simulink model "SimunlikReferenceDiffWindowSizes"  (R2021b)
settings: Solver=VariableStepAuto  StartTime=0.0  StopTime=2048*15/fs  RelTol=1e-3
InitFcn:
  | f = 12.288e6;
  | fs = 153.6e6;
  | N1 = 256;
  | N2 = 512;
  | N3 = 1024;
  | N4 = 2048;
  | N5 = 4096;
  | n1 = 0:N1-1;
  | n2 = 0:N2-1;
  | n3 = 0:N3-1;
  | n4 = 0:N4-1;
  | n5 = 0:N5-1;
  | Hamming1 = 0.54 - 0.46 * cos(2*pi*n1/N1);
  | Hamming2 = 0.54 - 0.46 * cos(2*pi*n2/N2);
  | Hamming3 = 0.54 - 0.46 * cos(2*pi*n3/N3);
  | Hamming4 = 0.54 - 0.46 * cos(2*pi*n4/N4);
  | Hamming5 = 0.54 - 0.46 * cos(2*pi*n5/N5);
  | Hanning1 = 0.5 * (1 + cos(2*pi*n1/N1));
  | Hanning2 = 0.5 * (1 + cos(2*pi*n2/N2));
  | Hanning3 = 0.5 * (1 + cos(2*pi*n3/N3));
  | Hanning4 = 0.5 * (1 + cos(2*pi*n4/N4));
  | Hanning5 = 0.5 * (1 + cos(2*pi*n5/N5));
  | Norm_Ham1 = sum(Hamming1);
  | Norm_Ham2 = sum(Hamming2);
  | Norm_Ham3 = sum(Hamming3);
  | Norm_Ham4 = sum(Hamming4);
  | Norm_Ham5 = sum(Hamming5);
  | Norm_Han1 = sum(Hanning1);
  | Norm_Han2 = sum(Hanning2);
  | Norm_Han3 = sum(Hanning3);
  | Norm_Han4 = sum(Hanning4);
  | Norm_Han5 = sum(Hanning5);
undefined symbols (not defined in the file): AXI4, Lite
libraries: dspxfrm3 x10, dspsigops x10, hdlBasic x7, hdlsllib x1, vmcUtilities x1
settings Model: Creator=yxb20126  LastModifiedBy=yxb20126

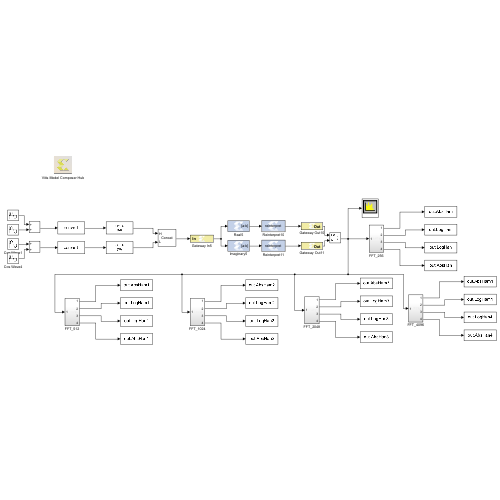
[thumbnail: Simulink's stored preview of the top-level diagram]
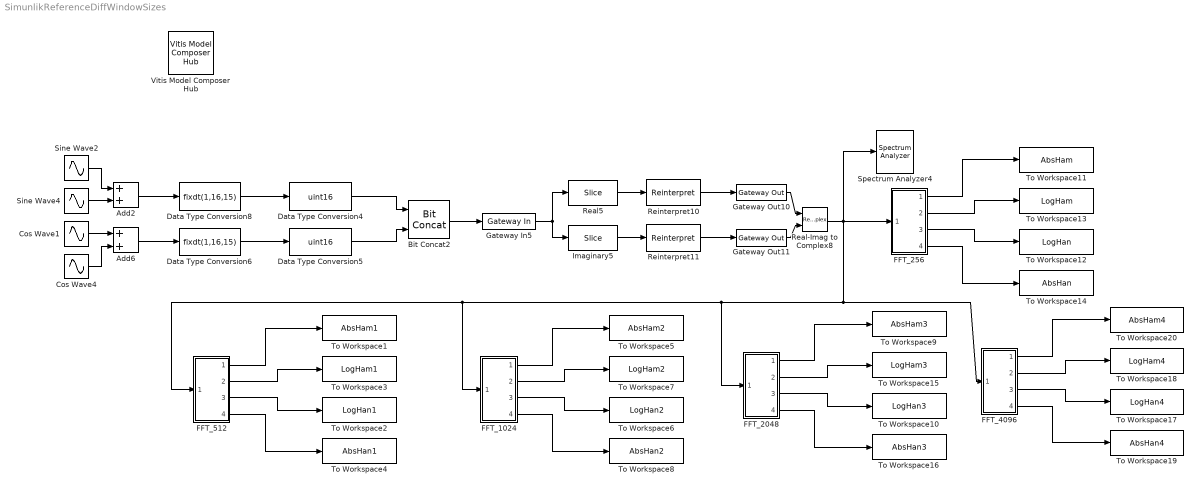
== system SimunlikReferenceDiffWindowSizes ==
  Add2 : Sum
  Add6 : Sum
  Bit Concat2 : hdlsllib/Logic and Bit Operations/Bit Concat  numInputs=2
  Cos Wave1 : Sin  Amplitude=0.4  Frequency=f*2*pi  Phase=pi/2  SampleTime=1/fs
  Cos Wave4 : Sin  Amplitude=0.4  Frequency=f*pi  Phase=pi/2  SampleTime=1/fs
  Data Type Conversion4 : DataTypeConversion  OutDataTypeStr=uint16  ConvertRealWorld=Stored Integer (SI)
  Data Type Conversion5 : DataTypeConversion  OutDataTypeStr=uint16  ConvertRealWorld=Stored Integer (SI)
  Data Type Conversion6 : DataTypeConversion  OutDataTypeStr=fixdt(1,16,15)  SaturateOnIntegerOverflow=on
  Data Type Conversion8 : DataTypeConversion  OutDataTypeStr=fixdt(1,16,15)  SaturateOnIntegerOverflow=on
  FFT_1024 : Subsystem
  FFT_2048 : Subsystem
  FFT_256 : Subsystem
  FFT_4096 : Subsystem
  FFT_512 : Subsystem
  Gateway In5 : hdlBasic/Gateway In  gui_display_data_type=Fixed-point  arith_type=Unsigned  n_bits=32  bin_pt=0  preci_type=Single  exp_width=8  frac_width=24  rows=1  columns=1  quantization=Truncate  overflow=Wrap  period=1/fs  UseAsADC=off  ADCChannel='1'  interface=AXI4-Lite  automatic_assignment=on  address_offset=hex2dec('00')  intf_name=''  intf_description=''  default_value=0  timing_constraint=None  locs_specified=off  LOCs={}  io_standard={}  inherit_from_input=off  hdl_port=on  XmcBlockStatus=1  maskContainerNames=group4  block_type=gatewayin  block_config=sysgen:gateway_in_config  block_width_w=590  block_height_w=620  block_width=640  block_height=850
  Gateway Out10 : hdlBasic/Gateway Out  inherit_from_input=off  hdl_port=on  rows=1  columns=1  UseAsDAC=off  DACChannel='1'  interface=AXI4-Lite  automatic_assignment=on  address_offset=hex2dec('00')  intf_name=''  intf_description=''  timing_constraint=None  locs_specified=off  LOCs={}  io_standard={}  XmcBlockStatus=1  maskContainerNames=group4  block_type=gatewayout  block_config=sysgen:gateway_out_config  block_width_w=590  block_height_w=620  block_width=620  block_height=750
  Gateway Out11 : hdlBasic/Gateway Out  inherit_from_input=off  hdl_port=on  rows=1  columns=1  UseAsDAC=off  DACChannel='1'  interface=AXI4-Lite  automatic_assignment=on  address_offset=hex2dec('00')  intf_name=''  intf_description=''  timing_constraint=None  locs_specified=off  LOCs={}  io_standard={}  XmcBlockStatus=1  maskContainerNames=group4  block_type=gatewayout  block_config=sysgen:gateway_out_config  block_width_w=590  block_height_w=620  block_width=620  block_height=750
  Imaginary5 : hdlBasic/Slice  nbits=16  boolean_output=off  mode=Two Bit Locations  bit1=31  base1=LSB of Input  bit0=16  base0=LSB of Input  XmcBlockStatus=1  maskContainerNames=group1  block_type=slice  block_config=sysgen:Slice_config
  Real-Imag to Complex8 : RealImagToComplex
  Real5 : hdlBasic/Slice  nbits=16  boolean_output=off  mode=Two Bit Locations  bit1=15  base1=LSB of Input  bit0=0  base0=LSB of Input  XmcBlockStatus=1  maskContainerNames=group1  block_type=slice  block_config=sysgen:Slice_config
  Reinterpret10 : hdlBasic/Reinterpret  force_arith_type=on  arith_type="Signed  (2's comp)"  force_bin_pt=off  bin_pt=0  XmcBlockStatus=1  maskContainerNames=group1  block_type=reinterpret  block_config=sysgen:Reinterpret_config
  Reinterpret11 : hdlBasic/Reinterpret  force_arith_type=on  arith_type="Signed  (2's comp)"  force_bin_pt=off  bin_pt=0  XmcBlockStatus=1  maskContainerNames=group1  block_type=reinterpret  block_config=sysgen:Reinterpret_config
  Sine Wave2 : Sin  Amplitude=0.4  Frequency=f*2*pi  SampleTime=1/fs
  Sine Wave4 : Sin  Amplitude=0.4  Frequency=f*pi  SampleTime=1/fs
  Spectrum Analyzer4 : SpectrumAnalyzer
  To Workspace1 : ToWorkspace  VariableName=AbsHam1  SampleTime=-1
      settings: Save2DSignal=2-D array (concatenate along first dimension)
  To Workspace10 : ToWorkspace  VariableName=LogHan3  SampleTime=-1
      settings: Save2DSignal=2-D array (concatenate along first dimension)
  To Workspace11 : ToWorkspace  VariableName=AbsHam  SampleTime=-1
      settings: Save2DSignal=2-D array (concatenate along first dimension)
  To Workspace12 : ToWorkspace  VariableName=LogHan  SampleTime=-1
      settings: Save2DSignal=2-D array (concatenate along first dimension)
  To Workspace13 : ToWorkspace  VariableName=LogHam  SampleTime=-1
      settings: Save2DSignal=2-D array (concatenate along first dimension)
  To Workspace14 : ToWorkspace  VariableName=AbsHan  SampleTime=-1
      settings: Save2DSignal=2-D array (concatenate along first dimension)
  To Workspace15 : ToWorkspace  VariableName=LogHam3  SampleTime=-1
      settings: Save2DSignal=2-D array (concatenate along first dimension)
  To Workspace16 : ToWorkspace  VariableName=AbsHan3  SampleTime=-1
      settings: Save2DSignal=2-D array (concatenate along first dimension)
  To Workspace17 : ToWorkspace  VariableName=LogHan4  SampleTime=-1
      settings: Save2DSignal=2-D array (concatenate along first dimension)
  To Workspace18 : ToWorkspace  VariableName=LogHam4  SampleTime=-1
      settings: Save2DSignal=2-D array (concatenate along first dimension)
  To Workspace19 : ToWorkspace  VariableName=AbsHan4  SampleTime=-1
      settings: Save2DSignal=2-D array (concatenate along first dimension)
  To Workspace2 : ToWorkspace  VariableName=LogHan1  SampleTime=-1
      settings: Save2DSignal=2-D array (concatenate along first dimension)
  To Workspace20 : ToWorkspace  VariableName=AbsHam4  SampleTime=-1
      settings: Save2DSignal=2-D array (concatenate along first dimension)
  To Workspace3 : ToWorkspace  VariableName=LogHam1  SampleTime=-1
      settings: Save2DSignal=2-D array (concatenate along first dimension)
  To Workspace4 : ToWorkspace  VariableName=AbsHan1  SampleTime=-1
      settings: Save2DSignal=2-D array (concatenate along first dimension)
  To Workspace5 : ToWorkspace  VariableName=AbsHam2  SampleTime=-1
      settings: Save2DSignal=2-D array (concatenate along first dimension)
  To Workspace6 : ToWorkspace  VariableName=LogHan2  SampleTime=-1
      settings: Save2DSignal=2-D array (concatenate along first dimension)
  To Workspace7 : ToWorkspace  VariableName=LogHam2  SampleTime=-1
      settings: Save2DSignal=2-D array (concatenate along first dimension)
  To Workspace8 : ToWorkspace  VariableName=AbsHan2  SampleTime=-1
      settings: Save2DSignal=2-D array (concatenate along first dimension)
  To Workspace9 : ToWorkspace  VariableName=AbsHam3  SampleTime=-1
      settings: Save2DSignal=2-D array (concatenate along first dimension)
  Vitis Model Composer Hub : vmcUtilities/Vitis Model Composer Hub  Tag=genX  CodeGeneration=off  SubsystemName=<enter or select subsystem name>  TargetDirectory=./code  ExportType=HLS C++ code  IpVendor=xilinx.com  IpLibrary=hls  IpVersion=1.0  IpHWLanguage=Verilog  AieCompilerOptions={}  CreateTestbench=off  TestbenchStackSize=10  RunAieSim=off  AieSimTimeout=50000  RunAieSimProfiling=off  LaunchVitisAnalyzer=off  PlotOutput=off  RunX86Sim=off  X86SimTimeout=10  GenHwImage=off  PlatformType=Not Specified  HwSystemType=Baremetal  HwValidationTarget=hw  ProjDevice=xczu48dr-ffvg1517-2-e  ProjDevicePart=xczu48dr-ffvg1517-2-e  SamplePeriod=-1  ClockFrequency=200  DataPathParallelism=1  xilinxfamily=zynquplusRFSOC  part=xczu48dr  speed=-2-e  package=ffvg1517  directory=./netlist  testbench=off  incr_netlist=off  synthesis_tool=Vivado  clock_wrapper=Clock Enables  dbl_ovrd=According to Block Masks  dcm_input_clock_period=10  sysclk_period=(1/fs)*10e9  simulink_period=1/fs  eval_field=0
  wires:
  FFT_256/1(Out1) -> To Workspace11/1
  FFT_256/2(Out2) -> To Workspace13/1
  Gateway Out10/1 -> Real-Imag to Complex8/1
  FFT_256/4(Out4) -> To Workspace14/1
  FFT_256/3(Out3) -> To Workspace12/1
  Reinterpret11/1 -> Gateway Out11/1
  Real-Imag to Complex8/1 -> FFT_4096/1(In1), FFT_2048/1(In1), FFT_1024/1(In1), FFT_512/1(In1), FFT_256/1(In1), Spectrum Analyzer4/1
  Gateway In5/1 -> Imaginary5/1, Real5/1
  Imaginary5/1 -> Reinterpret11/1
  Reinterpret10/1 -> Gateway Out10/1
  Gateway Out11/1 -> Real-Imag to Complex8/2
  Real5/1 -> Reinterpret10/1
  FFT_512/3(Out3) -> To Workspace2/1
  FFT_512/4(Out4) -> To Workspace4/1
  FFT_512/2(Out2) -> To Workspace3/1
  FFT_512/1(Out1) -> To Workspace1/1
  FFT_1024/1(Out1) -> To Workspace5/1
  FFT_1024/2(Out2) -> To Workspace7/1
  FFT_1024/4(Out4) -> To Workspace8/1
  FFT_1024/3(Out3) -> To Workspace6/1
  FFT_2048/3(Out3) -> To Workspace10/1
  FFT_2048/4(Out4) -> To Workspace16/1
  FFT_2048/2(Out2) -> To Workspace15/1
  FFT_2048/1(Out1) -> To Workspace9/1
  FFT_4096/1(Out1) -> To Workspace20/1
  FFT_4096/2(Out2) -> To Workspace18/1
  FFT_4096/4(Out4) -> To Workspace19/1
  FFT_4096/3(Out3) -> To Workspace17/1
  Data Type Conversion5/1 -> Bit Concat2/2
  Data Type Conversion8/1 -> Data Type Conversion4/1
  Add6/1 -> Data Type Conversion6/1
  Sine Wave4/1 -> Add2/2
  Sine Wave2/1 -> Add2/1
  Add2/1 -> Data Type Conversion8/1
  Cos Wave1/1 -> Add6/1
  Data Type Conversion6/1 -> Data Type Conversion5/1
  Data Type Conversion4/1 -> Bit Concat2/1
  Cos Wave4/1 -> Add6/2
  Bit Concat2/1 -> Gateway In5/1

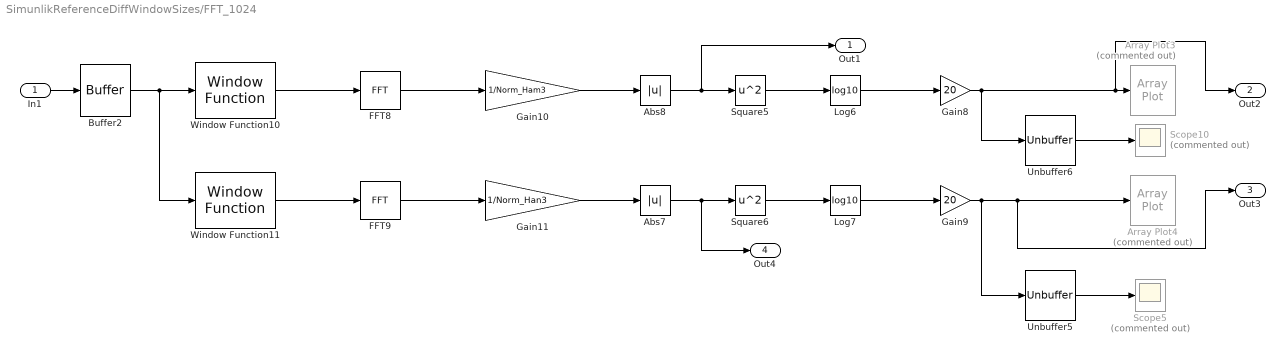
== system SimunlikReferenceDiffWindowSizes/FFT_1024 ==
  In1 : Inport
  Abs7 : Abs
  Abs8 : Abs
  Array Plot3 : ArrayPlot  Commented=on  WindowPosition=[827.000000,398.000000,581.000000,481.000000,]  YLimits=[-59.68956955456875,167.07325575587276]  ShowLegend=on
  Array Plot4 : ArrayPlot  Commented=on  WindowPosition=[214.000000,393.000000,581.000000,481.000000,]  YLimits=[-59.68956955456875,167.07325575587276]  ShowLegend=on
  Buffer2 : Buffer  N=N3  OutputFrames=off
  FFT8 : dspxfrm3/FFT  FFTImplementation=Auto  CompMethod=Table lookup  TableOpt=NEW  TableOptActive=Speed  BitRevOrder=off  Normalize=off  InheritFFTLength=off  FFTLength=N3  WrapInput=off  roundingMode=Floor  overflowMode=off  firstCoeffDataTypeStr=Inherit: Same word length as input  firstCoeffLastDataTypeStr=Inherit: Same word length as input  outputMin=[]  outputMax=[]
  FFT9 : dspxfrm3/FFT  FFTImplementation=Auto  CompMethod=Table lookup  TableOpt=NEW  TableOptActive=Speed  BitRevOrder=off  Normalize=off  InheritFFTLength=off  FFTLength=N3  WrapInput=off  roundingMode=Floor  overflowMode=off  firstCoeffDataTypeStr=Inherit: Same word length as input  firstCoeffLastDataTypeStr=Inherit: Same word length as input  outputMin=[]  outputMax=[]
  Gain10 : Gain  Gain=1/Norm_Ham3
  Gain11 : Gain  Gain=1/Norm_Han3
  Gain8 : Gain  Gain=20
  Gain9 : Gain  Gain=20
  Log6 : Math  Operator=log10  OutputSignalType=complex  SaturateOnIntegerOverflow=on
  Log7 : Math  Operator=log10  OutputSignalType=complex  SaturateOnIntegerOverflow=on
  Scope10 : Scope  Commented=on
  Scope5 : Scope  Commented=on
  Square5 : Math  Operator=square  SaturateOnIntegerOverflow=on
  Square6 : Math  Operator=square  SaturateOnIntegerOverflow=on
  Unbuffer5 : Unbuffer
  Unbuffer6 : Unbuffer
  Window Function10 : dspsigops/Window Function  winmode=Apply window to input  wintype=Hamming  sampmode=Continuous  samptime=1  N=64  Rs=50  beta=10  winsamp=Symmetric  UserWindow=hamming  OptParams=off  UserParams={'symmetric'}  dataType=double  isSigned=on  wordLen=16  udDataType=sfix(16)  fracBitsMode=Best precision  numFracBits=15  roundingMode=Floor  overflowMode=on  numSidelobes=4  sidelobeLevel=-30
      settings: SourceProductBaseCode=DS
  Window Function11 : dspsigops/Window Function  winmode=Apply window to input  wintype=Hann  sampmode=Continuous  samptime=1  N=64  Rs=50  beta=10  winsamp=Symmetric  UserWindow=hamming  OptParams=off  UserParams={'symmetric'}  dataType=double  isSigned=on  wordLen=16  udDataType=sfix(16)  fracBitsMode=Best precision  numFracBits=15  roundingMode=Floor  overflowMode=on  numSidelobes=4  sidelobeLevel=-30
      settings: SourceProductBaseCode=DS
  Out1 : Outport
  Out2 : Outport  Port=2
  Out3 : Outport  Port=3
  Out4 : Outport  Port=4
  wires:
  FFT8/1 -> Gain10/1
  Unbuffer6/1 -> Scope10/1
  Log6/1 -> Gain8/1
  Gain8/1 -> Out2/1, Array Plot3/1, Unbuffer6/1
  Square5/1 -> Log6/1
  Gain9/1 -> Out3/1, Array Plot4/1, Unbuffer5/1
  Buffer2/1 -> Window Function11/1, Window Function10/1
  Abs8/1 -> Out1/1, Square5/1
  Window Function11/1 -> FFT9/1
  Log7/1 -> Gain9/1
  Square6/1 -> Log7/1
  Window Function10/1 -> FFT8/1
  Unbuffer5/1 -> Scope5/1
  In1/1 -> Buffer2/1
  Abs7/1 -> Out4/1, Square6/1
  Gain10/1 -> Abs8/1
  Gain11/1 -> Abs7/1
  FFT9/1 -> Gain11/1

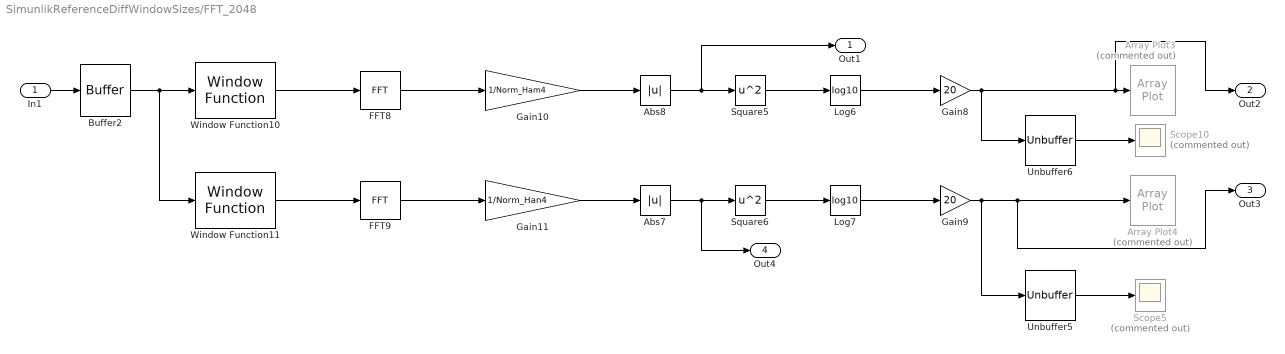
== system SimunlikReferenceDiffWindowSizes/FFT_2048 ==
  In1 : Inport
  Abs7 : Abs
  Abs8 : Abs
  Array Plot3 : ArrayPlot  Commented=on  WindowPosition=[827.000000,398.000000,581.000000,481.000000,]  YLimits=[-59.68956955456875,167.07325575587276]  ShowLegend=on
  Array Plot4 : ArrayPlot  Commented=on  WindowPosition=[214.000000,393.000000,581.000000,481.000000,]  YLimits=[-59.68956955456875,167.07325575587276]  ShowLegend=on
  Buffer2 : Buffer  N=N4  OutputFrames=off
  FFT8 : dspxfrm3/FFT  FFTImplementation=Auto  CompMethod=Table lookup  TableOpt=NEW  TableOptActive=Speed  BitRevOrder=off  Normalize=off  InheritFFTLength=off  FFTLength=N4  WrapInput=off  roundingMode=Floor  overflowMode=off  firstCoeffDataTypeStr=Inherit: Same word length as input  firstCoeffLastDataTypeStr=Inherit: Same word length as input  outputMin=[]  outputMax=[]
  FFT9 : dspxfrm3/FFT  FFTImplementation=Auto  CompMethod=Table lookup  TableOpt=NEW  TableOptActive=Speed  BitRevOrder=off  Normalize=off  InheritFFTLength=off  FFTLength=N4  WrapInput=off  roundingMode=Floor  overflowMode=off  firstCoeffDataTypeStr=Inherit: Same word length as input  firstCoeffLastDataTypeStr=Inherit: Same word length as input  outputMin=[]  outputMax=[]
  Gain10 : Gain  Gain=1/Norm_Ham4
  Gain11 : Gain  Gain=1/Norm_Han4
  Gain8 : Gain  Gain=20
  Gain9 : Gain  Gain=20
  Log6 : Math  Operator=log10  OutputSignalType=complex  SaturateOnIntegerOverflow=on
  Log7 : Math  Operator=log10  OutputSignalType=complex  SaturateOnIntegerOverflow=on
  Scope10 : Scope  Commented=on
  Scope5 : Scope  Commented=on
  Square5 : Math  Operator=square  SaturateOnIntegerOverflow=on
  Square6 : Math  Operator=square  SaturateOnIntegerOverflow=on
  Unbuffer5 : Unbuffer
  Unbuffer6 : Unbuffer
  Window Function10 : dspsigops/Window Function  winmode=Apply window to input  wintype=Hamming  sampmode=Continuous  samptime=1  N=64  Rs=50  beta=10  winsamp=Symmetric  UserWindow=hamming  OptParams=off  UserParams={'symmetric'}  dataType=double  isSigned=on  wordLen=16  udDataType=sfix(16)  fracBitsMode=Best precision  numFracBits=15  roundingMode=Floor  overflowMode=on  numSidelobes=4  sidelobeLevel=-30
      settings: SourceProductBaseCode=DS
  Window Function11 : dspsigops/Window Function  winmode=Apply window to input  wintype=Hann  sampmode=Continuous  samptime=1  N=64  Rs=50  beta=10  winsamp=Symmetric  UserWindow=hamming  OptParams=off  UserParams={'symmetric'}  dataType=double  isSigned=on  wordLen=16  udDataType=sfix(16)  fracBitsMode=Best precision  numFracBits=15  roundingMode=Floor  overflowMode=on  numSidelobes=4  sidelobeLevel=-30
      settings: SourceProductBaseCode=DS
  Out1 : Outport
  Out2 : Outport  Port=2
  Out3 : Outport  Port=3
  Out4 : Outport  Port=4
  wires:
  FFT9/1 -> Gain11/1
  Gain11/1 -> Abs7/1
  Gain10/1 -> Abs8/1
  Abs7/1 -> Square6/1, Out4/1
  In1/1 -> Buffer2/1
  Unbuffer5/1 -> Scope5/1
  Window Function10/1 -> FFT8/1
  Square6/1 -> Log7/1
  Log7/1 -> Gain9/1
  Window Function11/1 -> FFT9/1
  Abs8/1 -> Square5/1, Out1/1
  Buffer2/1 -> Window Function10/1, Window Function11/1
  Gain9/1 -> Unbuffer5/1, Array Plot4/1, Out3/1
  Square5/1 -> Log6/1
  Gain8/1 -> Unbuffer6/1, Array Plot3/1, Out2/1
  Log6/1 -> Gain8/1
  Unbuffer6/1 -> Scope10/1
  FFT8/1 -> Gain10/1

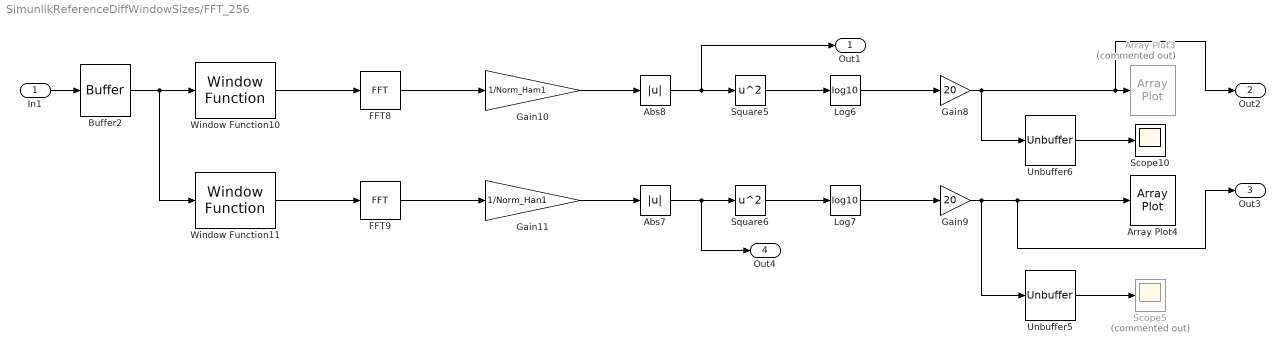
== system SimunlikReferenceDiffWindowSizes/FFT_256 ==
  In1 : Inport
  Abs7 : Abs
  Abs8 : Abs
  Array Plot3 : ArrayPlot  Commented=on  WindowPosition=[827.000000,398.000000,581.000000,481.000000,]  YLimits=[-59.68956955456875,167.07325575587276]  ShowLegend=on
  Array Plot4 : ArrayPlot  WindowPosition=[214.000000,393.000000,581.000000,481.000000,]  YLimits=[-59.68956955456875,167.07325575587276]  ShowLegend=on
  Buffer2 : Buffer  N=N1  OutputFrames=off
  FFT8 : dspxfrm3/FFT  FFTImplementation=Auto  CompMethod=Table lookup  TableOpt=NEW  TableOptActive=Speed  BitRevOrder=off  Normalize=off  InheritFFTLength=off  FFTLength=N1  WrapInput=off  roundingMode=Floor  overflowMode=off  firstCoeffDataTypeStr=Inherit: Same word length as input  firstCoeffLastDataTypeStr=Inherit: Same word length as input  outputMin=[]  outputMax=[]
  FFT9 : dspxfrm3/FFT  FFTImplementation=Auto  CompMethod=Table lookup  TableOpt=NEW  TableOptActive=Speed  BitRevOrder=off  Normalize=off  InheritFFTLength=off  FFTLength=N1  WrapInput=off  roundingMode=Floor  overflowMode=off  firstCoeffDataTypeStr=Inherit: Same word length as input  firstCoeffLastDataTypeStr=Inherit: Same word length as input  outputMin=[]  outputMax=[]
  Gain10 : Gain  Gain=1/Norm_Ham1
  Gain11 : Gain  Gain=1/Norm_Han1
  Gain8 : Gain  Gain=20
  Gain9 : Gain  Gain=20
  Log6 : Math  Operator=log10  OutputSignalType=complex  SaturateOnIntegerOverflow=on
  Log7 : Math  Operator=log10  OutputSignalType=complex  SaturateOnIntegerOverflow=on
  Scope10 : Scope
  Scope5 : Scope  Commented=on
  Square5 : Math  Operator=square  SaturateOnIntegerOverflow=on
  Square6 : Math  Operator=square  SaturateOnIntegerOverflow=on
  Unbuffer5 : Unbuffer
  Unbuffer6 : Unbuffer
  Window Function10 : dspsigops/Window Function  winmode=Apply window to input  wintype=Hamming  sampmode=Continuous  samptime=1  N=64  Rs=50  beta=10  winsamp=Symmetric  UserWindow=hamming  OptParams=off  UserParams={'symmetric'}  dataType=double  isSigned=on  wordLen=16  udDataType=sfix(16)  fracBitsMode=Best precision  numFracBits=15  roundingMode=Floor  overflowMode=on  numSidelobes=4  sidelobeLevel=-30
      settings: SourceProductBaseCode=DS
  Window Function11 : dspsigops/Window Function  winmode=Apply window to input  wintype=Hann  sampmode=Continuous  samptime=1  N=64  Rs=50  beta=10  winsamp=Symmetric  UserWindow=hamming  OptParams=off  UserParams={'symmetric'}  dataType=double  isSigned=on  wordLen=16  udDataType=sfix(16)  fracBitsMode=Best precision  numFracBits=15  roundingMode=Floor  overflowMode=on  numSidelobes=4  sidelobeLevel=-30
      settings: SourceProductBaseCode=DS
  Out1 : Outport
  Out2 : Outport  Port=2
  Out3 : Outport  Port=3
  Out4 : Outport  Port=4
  wires:
  FFT8/1 -> Gain10/1
  Unbuffer6/1 -> Scope10/1
  Log6/1 -> Gain8/1
  Gain8/1 -> Out2/1, Array Plot3/1, Unbuffer6/1
  Square5/1 -> Log6/1
  Gain9/1 -> Out3/1, Array Plot4/1, Unbuffer5/1
  Buffer2/1 -> Window Function11/1, Window Function10/1
  Abs8/1 -> Out1/1, Square5/1
  Window Function11/1 -> FFT9/1
  Log7/1 -> Gain9/1
  Square6/1 -> Log7/1
  Window Function10/1 -> FFT8/1
  Unbuffer5/1 -> Scope5/1
  In1/1 -> Buffer2/1
  Abs7/1 -> Out4/1, Square6/1
  Gain10/1 -> Abs8/1
  Gain11/1 -> Abs7/1
  FFT9/1 -> Gain11/1

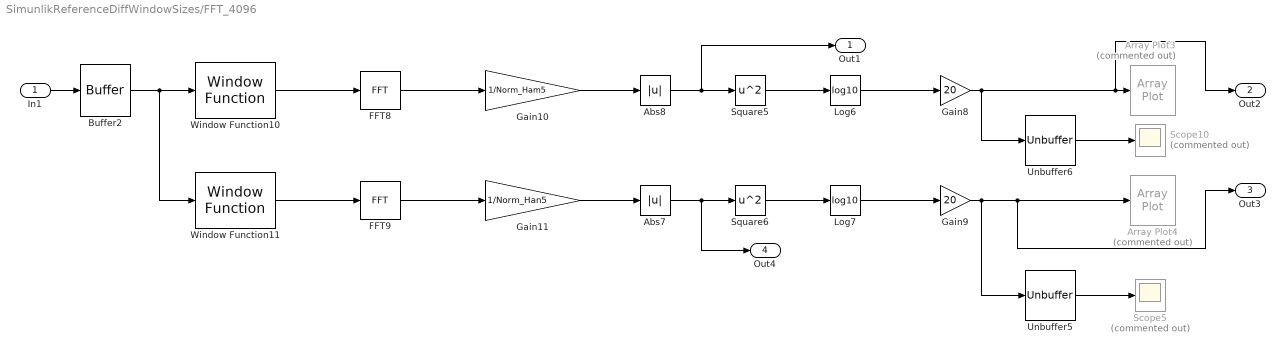
== system SimunlikReferenceDiffWindowSizes/FFT_4096 ==
  In1 : Inport
  Abs7 : Abs
  Abs8 : Abs
  Array Plot3 : ArrayPlot  Commented=on  WindowPosition=[827.000000,398.000000,581.000000,481.000000,]  YLimits=[-59.68956955456875,167.07325575587276]  ShowLegend=on
  Array Plot4 : ArrayPlot  Commented=on  WindowPosition=[214.000000,393.000000,581.000000,481.000000,]  YLimits=[-59.68956955456875,167.07325575587276]  ShowLegend=on
  Buffer2 : Buffer  N=N5  OutputFrames=off
  FFT8 : dspxfrm3/FFT  FFTImplementation=Auto  CompMethod=Table lookup  TableOpt=NEW  TableOptActive=Speed  BitRevOrder=off  Normalize=off  InheritFFTLength=off  FFTLength=N5  WrapInput=off  roundingMode=Floor  overflowMode=off  firstCoeffDataTypeStr=Inherit: Same word length as input  firstCoeffLastDataTypeStr=Inherit: Same word length as input  outputMin=[]  outputMax=[]
  FFT9 : dspxfrm3/FFT  FFTImplementation=Auto  CompMethod=Table lookup  TableOpt=NEW  TableOptActive=Speed  BitRevOrder=off  Normalize=off  InheritFFTLength=off  FFTLength=N5  WrapInput=off  roundingMode=Floor  overflowMode=off  firstCoeffDataTypeStr=Inherit: Same word length as input  firstCoeffLastDataTypeStr=Inherit: Same word length as input  outputMin=[]  outputMax=[]
  Gain10 : Gain  Gain=1/Norm_Ham5
  Gain11 : Gain  Gain=1/Norm_Han5
  Gain8 : Gain  Gain=20
  Gain9 : Gain  Gain=20
  Log6 : Math  Operator=log10  OutputSignalType=complex  SaturateOnIntegerOverflow=on
  Log7 : Math  Operator=log10  OutputSignalType=complex  SaturateOnIntegerOverflow=on
  Scope10 : Scope  Commented=on
  Scope5 : Scope  Commented=on
  Square5 : Math  Operator=square  SaturateOnIntegerOverflow=on
  Square6 : Math  Operator=square  SaturateOnIntegerOverflow=on
  Unbuffer5 : Unbuffer
  Unbuffer6 : Unbuffer
  Window Function10 : dspsigops/Window Function  winmode=Apply window to input  wintype=Hamming  sampmode=Continuous  samptime=1  N=64  Rs=50  beta=10  winsamp=Symmetric  UserWindow=hamming  OptParams=off  UserParams={'symmetric'}  dataType=double  isSigned=on  wordLen=16  udDataType=sfix(16)  fracBitsMode=Best precision  numFracBits=15  roundingMode=Floor  overflowMode=on  numSidelobes=4  sidelobeLevel=-30
      settings: SourceProductBaseCode=DS
  Window Function11 : dspsigops/Window Function  winmode=Apply window to input  wintype=Hann  sampmode=Continuous  samptime=1  N=64  Rs=50  beta=10  winsamp=Symmetric  UserWindow=hamming  OptParams=off  UserParams={'symmetric'}  dataType=double  isSigned=on  wordLen=16  udDataType=sfix(16)  fracBitsMode=Best precision  numFracBits=15  roundingMode=Floor  overflowMode=on  numSidelobes=4  sidelobeLevel=-30
      settings: SourceProductBaseCode=DS
  Out1 : Outport
  Out2 : Outport  Port=2
  Out3 : Outport  Port=3
  Out4 : Outport  Port=4
  wires:
  FFT8/1 -> Gain10/1
  Unbuffer6/1 -> Scope10/1
  Log6/1 -> Gain8/1
  Gain8/1 -> Out2/1, Array Plot3/1, Unbuffer6/1
  Square5/1 -> Log6/1
  Gain9/1 -> Out3/1, Array Plot4/1, Unbuffer5/1
  Buffer2/1 -> Window Function11/1, Window Function10/1
  Abs8/1 -> Out1/1, Square5/1
  Window Function11/1 -> FFT9/1
  Log7/1 -> Gain9/1
  Square6/1 -> Log7/1
  Window Function10/1 -> FFT8/1
  Unbuffer5/1 -> Scope5/1
  In1/1 -> Buffer2/1
  Abs7/1 -> Out4/1, Square6/1
  Gain10/1 -> Abs8/1
  Gain11/1 -> Abs7/1
  FFT9/1 -> Gain11/1

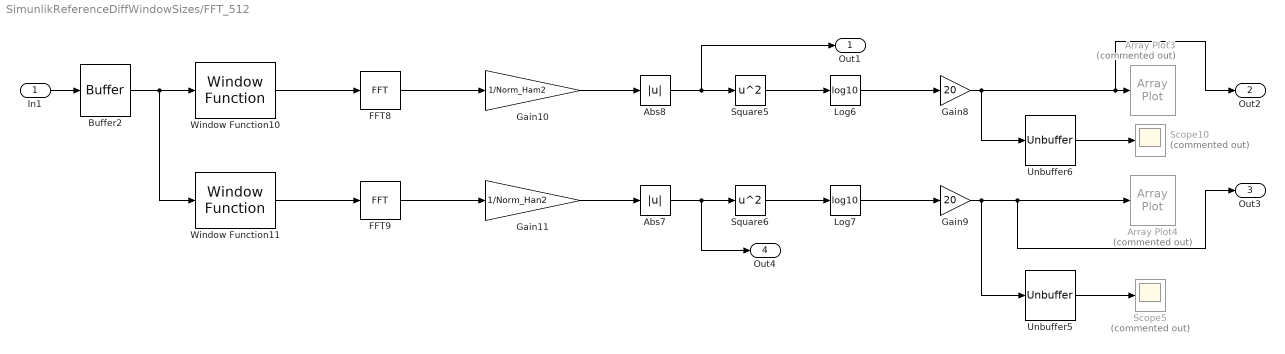
== system SimunlikReferenceDiffWindowSizes/FFT_512 ==
  In1 : Inport
  Abs7 : Abs
  Abs8 : Abs
  Array Plot3 : ArrayPlot  Commented=on  WindowPosition=[827.000000,398.000000,581.000000,481.000000,]  YLimits=[-59.68956955456875,167.07325575587276]  ShowLegend=on
  Array Plot4 : ArrayPlot  Commented=on  WindowPosition=[214.000000,393.000000,581.000000,481.000000,]  YLimits=[-59.68956955456875,167.07325575587276]  ShowLegend=on
  Buffer2 : Buffer  N=N2  OutputFrames=off
  FFT8 : dspxfrm3/FFT  FFTImplementation=Auto  CompMethod=Table lookup  TableOpt=NEW  TableOptActive=Speed  BitRevOrder=off  Normalize=off  InheritFFTLength=off  FFTLength=N2  WrapInput=off  roundingMode=Floor  overflowMode=off  firstCoeffDataTypeStr=Inherit: Same word length as input  firstCoeffLastDataTypeStr=Inherit: Same word length as input  outputMin=[]  outputMax=[]
  FFT9 : dspxfrm3/FFT  FFTImplementation=Auto  CompMethod=Table lookup  TableOpt=NEW  TableOptActive=Speed  BitRevOrder=off  Normalize=off  InheritFFTLength=off  FFTLength=N2  WrapInput=off  roundingMode=Floor  overflowMode=off  firstCoeffDataTypeStr=Inherit: Same word length as input  firstCoeffLastDataTypeStr=Inherit: Same word length as input  outputMin=[]  outputMax=[]
  Gain10 : Gain  Gain=1/Norm_Ham2
  Gain11 : Gain  Gain=1/Norm_Han2
  Gain8 : Gain  Gain=20
  Gain9 : Gain  Gain=20
  Log6 : Math  Operator=log10  OutputSignalType=complex  SaturateOnIntegerOverflow=on
  Log7 : Math  Operator=log10  OutputSignalType=complex  SaturateOnIntegerOverflow=on
  Scope10 : Scope  Commented=on
  Scope5 : Scope  Commented=on
  Square5 : Math  Operator=square  SaturateOnIntegerOverflow=on
  Square6 : Math  Operator=square  SaturateOnIntegerOverflow=on
  Unbuffer5 : Unbuffer
  Unbuffer6 : Unbuffer
  Window Function10 : dspsigops/Window Function  winmode=Apply window to input  wintype=Hamming  sampmode=Continuous  samptime=1  N=64  Rs=50  beta=10  winsamp=Symmetric  UserWindow=hamming  OptParams=off  UserParams={'symmetric'}  dataType=double  isSigned=on  wordLen=16  udDataType=sfix(16)  fracBitsMode=Best precision  numFracBits=15  roundingMode=Floor  overflowMode=on  numSidelobes=4  sidelobeLevel=-30
      settings: SourceProductBaseCode=DS
  Window Function11 : dspsigops/Window Function  winmode=Apply window to input  wintype=Hann  sampmode=Continuous  samptime=1  N=64  Rs=50  beta=10  winsamp=Symmetric  UserWindow=hamming  OptParams=off  UserParams={'symmetric'}  dataType=double  isSigned=on  wordLen=16  udDataType=sfix(16)  fracBitsMode=Best precision  numFracBits=15  roundingMode=Floor  overflowMode=on  numSidelobes=4  sidelobeLevel=-30
      settings: SourceProductBaseCode=DS
  Out1 : Outport
  Out2 : Outport  Port=2
  Out3 : Outport  Port=3
  Out4 : Outport  Port=4
  wires:
  FFT9/1 -> Gain11/1
  Gain11/1 -> Abs7/1
  Gain10/1 -> Abs8/1
  Abs7/1 -> Square6/1, Out4/1
  In1/1 -> Buffer2/1
  Unbuffer5/1 -> Scope5/1
  Window Function10/1 -> FFT8/1
  Square6/1 -> Log7/1
  Log7/1 -> Gain9/1
  Window Function11/1 -> FFT9/1
  Abs8/1 -> Square5/1, Out1/1
  Buffer2/1 -> Window Function10/1, Window Function11/1
  Gain9/1 -> Unbuffer5/1, Array Plot4/1, Out3/1
  Square5/1 -> Log6/1
  Gain8/1 -> Unbuffer6/1, Array Plot3/1, Out2/1
  Log6/1 -> Gain8/1
  Unbuffer6/1 -> Scope10/1
  FFT8/1 -> Gain10/1
